simulink model "MdXXStatCtrlHarness"  (R2018b)
settings: Solver=FixedStepDiscrete  StartTime=0.0  StopTime=10.0  FixedStep=0.01  RelTol=1e-3
settings Model: PauseTimes=0.05  Creator=sn2xws  LastModifiedBy=sn2xws

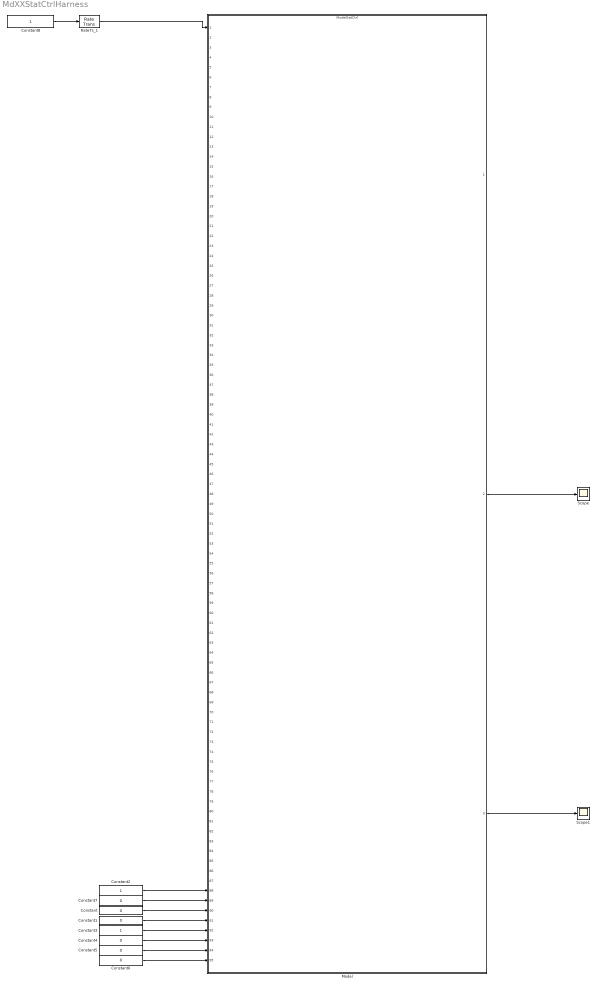
== system MdXXStatCtrlHarness ==
  Constant : Constant  Value=0  OutDataTypeStr=uint16
  Constant1 : Constant  Value=0  OutDataTypeStr=uint16
  Constant2 : Constant  OutDataTypeStr=boolean
  Constant3 : Constant  OutDataTypeStr=boolean
  Constant{4..7} (4 alike) : Constant  Value=0  OutDataTypeStr=boolean
  Constant8 : Constant  OutDataTypeStr=boolean
  Model : ModelReference  ModelNameDialog=ModeStatCtrl.slx  SimulationMode=Normal  ModelReferenceVersion=1.81
  RateTs_1 : RateTransition
  Scope : Scope
  Scope1 : Scope
  wires:
  Constant/1 -> Model/90
  Constant1/1 -> Model/91
  Constant2/1 -> Model/88
  Model/2 -> Scope/1
  Constant3/1 -> Model/92
  Constant4/1 -> Model/93
  Constant5/1 -> Model/94
  Constant6/1 -> Model/95
  Constant7/1 -> Model/89
  Constant8/1 -> RateTs_1/1
  RateTs_1/1 -> Model/1
  Model/3 -> Scope1/1
